simulink model "CruiseControl_PI"  (R2018b)
settings: Solver=ode45  StartTime=0.0  StopTime=40.0  MaxStep=1e-2  RelTol=1e-3
values from neighbouring files (symbols this model uses):
  a = 200    [CruiseControl_param.m]    (also in Example_VehicleSteering_PP.m = 2)
  b = 10000    [CruiseControl_param.m]    (also in Example_VehicleSteering_PP.m = 4)
  g = 9.82    [CruiseControl_param.m]
  ki = 0.07    [CruiseControl_param.m]
  kp = 0.1    [CruiseControl_param.m]
  m = 1000    [CruiseControl_param.m]
settings Model: Creator=jofr  LastModifiedBy=sofiato
settings DataIOCC: LimitDataPoints=on  SaveFormat=Array  SignalLoggingSaveFormat=ModelDataLogs
settings OptimizationCC: BlockReduction=off  BooleanDataType=off  LifeSpan=inf
settings DebuggingCC: SaveWithParameterizedLinksMsg=none  UnderspecifiedInitializationDetection=Classic  MergeDetectMultiDrivingBlocksExec=none  SignalResolutionControl=TryResolveAllWithWarning  MultiTaskDSMMsg=warning  MultiTaskCondExecSysMsg=none  SFUnexpectedBacktrackingDiag=warning  SFNoUnconditionalDefaultTransitionDiag=warning  SFExecutionAtInitializationDiag=none
settings HardwareCC: ProdBitPerPointer=32  ProdBitPerSizeT=32  ProdBitPerPtrDiffT=32  ProdLargestAtomicFloat=None  ProdIntDivRoundTo=Undefined  ProdEndianess=Unspecified  ProdWordSize=32  ProdHWDeviceType=32-bit Generic  TargetUnknown=on
settings ModelReferenceCC: PropagateSignalLabelsOutOfModel=off
settings SFSimCC: SimUseLocalCustomCode=off
settings RTWCC: RTWUseLocalCustomCode=off
settings CodeAppCC: StateflowObjectComments=on
settings GRTTargetCC: TargetLangStandard=C89/C90 (ANSI)  GeneratePreprocessorConditionals=Disable all
settings ConfigComp: CovMetricSettings=dw  CovHtmlReporting=on  CovSaveCumulativeToWorkspaceVar=on  CovSaveSingleToWorkspaceVar=on  CovExternalEMLEnable=off

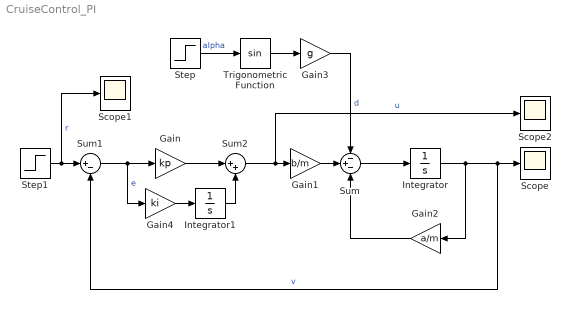
== system CruiseControl_PI ==
  Gain : Gain  Gain=kp
  Gain1 : Gain  Gain=b/m
  Gain2 : Gain  Gain=a/m
  Gain3 : Gain  Gain=g
  Gain4 : Gain  Gain=ki
  Integrator : Integrator  InitialCondition=25
  Integrator1 : Integrator
  Scope : Scope
  Scope1 : Scope
  Scope2 : Scope
  Step : Step  Time=1000  After=0.1  SampleTime=0
  Step1 : Step  Time=20  Before=25  After=30  SampleTime=0
  Sum : Sum  Inputs=-+-
  Sum1 : Sum  Inputs=|+-
  Sum2 : Sum  Inputs=|++
  Trigonometric Function : Trigonometry
  wires:
  Gain2/1 -> Sum/3
  Gain1/1 -> Sum/2
  Trigonometric Function/1 -> Gain3/1
  Sum/1 -> Integrator/1
  Step/1 -> Trigonometric Function/1  "alpha"
  Integrator/1 -> Scope/1, Sum1/2, Gain2/1  "v"
  Gain3/1 -> Sum/1  "d"
  Sum1/1 -> Gain4/1, Gain/1  "e"
  Step1/1 -> Scope1/1, Sum1/1  "r"
  Sum2/1 -> Scope2/1, Gain1/1  "u"
  Gain/1 -> Sum2/1
  Gain4/1 -> Integrator1/1
  Integrator1/1 -> Sum2/2
